simulink model "SimuMCC_LK"  (R2017b)
settings: Solver=VariableStepAuto  StartTime=0.0  StopTime=Tf  MaxStep=1e-4  RelTol=1e-3
values from neighbouring files (symbols this model uses):
  C0 = 0.0    (= 0)    [DataMCCEchant.m]
  Cl = 0    [DataMCCEchant.m]
  F = 0.0001    [DataMCCEchant.m]
  J = 2.20e-4    (= 0.00022)    [DataMCCEchant.m]
  Kelec = -place(Ae,Be,Pole_elec_desiree)    [DataMCCEchant.m]
  Kmeca = place(Am,Bm,Pole_meca_desiree)    [DataMCCEchant.m]
  Kphi = 0.061    [DataMCCEchant.m]
  L = 2.7e-3    (= 0.0027)    [DataMCCEchant.m]
  R = 1.22    [DataMCCEchant.m]
  Ts = 1e-4    (= 0.0001)    [DataMCCEchant.m]
undefined symbols (not defined in the file or in its folder): Cg, Commande, Fg, Gg, Ggi, KPi, KPw, TIi, TIw
settings Model: Creator=romaindelpoux  LastModifiedBy=Lubin Kerhuel
settings SolverCC: ZeroCrossControl=DisableAll

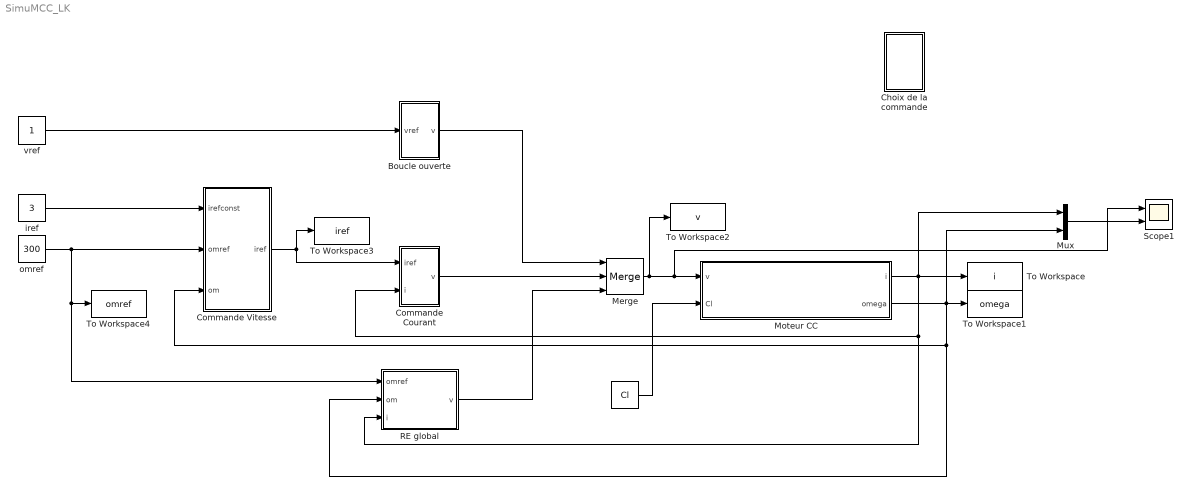
== system SimuMCC_LK ==
  " " : Constant  Value=Cl
  Boucle ouverte : Subsystem
  Choix de la commande : Subsystem
  Commande Courant : Subsystem
  Commande Vitesse : Subsystem
  Merge : Merge  Inputs=3
  Moteur CC : Subsystem
  Mux : Mux  Inputs=2
  RE global : Subsystem
  Scope1 : Scope  NumInputPorts=2
  To Workspace : ToWorkspace  VariableName=i  SaveFormat=Timeseries  SampleTime=-1
  To Workspace1 : ToWorkspace  VariableName=omega  SaveFormat=Timeseries  SampleTime=-1
  To Workspace2 : ToWorkspace  VariableName=v  SaveFormat=Timeseries  SampleTime=-1
  To Workspace3 : ToWorkspace  VariableName=iref  SaveFormat=Timeseries  SampleTime=-1
  To Workspace4 : ToWorkspace  VariableName=omref  SaveFormat=Timeseries  SampleTime=-1
  iref : Constant  Value=3
  omref : Constant  Value=300
  vref : Constant
  wires:
  Merge/1 -> To Workspace2/1, Scope1/1, Moteur CC/1(v)
  Moteur CC/2(omega) -> Mux/2, To Workspace1/1, RE global/2(om), Commande Vitesse/3(om)
  Moteur CC/1(i) -> Mux/1, RE global/3(i), Commande Courant/2(i), To Workspace/1
  omref/1 -> RE global/1(omref), To Workspace4/1, Commande Vitesse/2(omref)
  Commande Courant/1(v) -> Merge/2
  Commande Vitesse/1(iref) -> Commande Courant/1(iref), To Workspace3/1
  " "/1 -> Moteur CC/2(Cl)
  iref/1 -> Commande Vitesse/1(irefconst)
  vref/1 -> Boucle ouverte/1(vref)
  Boucle ouverte/1(v) -> Merge/1
  RE global/1(v) -> Merge/3
  Mux/1 -> Scope1/2

== system SimuMCC_LK/Boucle ouverte ==
  vref : Inport
  BO : Subsystem  TreatAsAtomicUnit=on
  v : Outport
  wires:
  BO/1(v) -> v/1
  vref/1 -> BO/1(vref)
  [BO] -> BO/Action

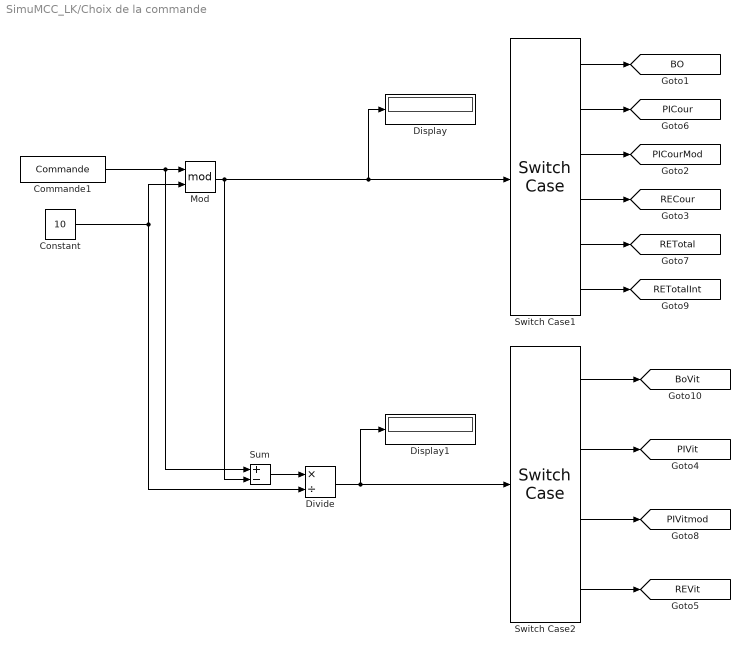
== system SimuMCC_LK/Choix de la commande ==
  Commande1 : Constant  Value=Commande
  Constant : Constant  Value=10
  Display : Display
  Display1 : Display
  Divide : Product  Inputs=*/
  Mod : Math  Operator=mod  SaturateOnIntegerOverflow=on
  Sum : Sum  Inputs=+-
  Switch Case1 : SwitchCase  CaseConditions={0, 1,2,3,4,5}  ShowDefaultCase=off
  Switch Case2 : SwitchCase  CaseConditions={0,1,2,3}  ShowDefaultCase=off
  tag scope: BO=global, BoVit=global, PICour=global, PICourMod=global, PIVit=global, PIVitmod=global, RECour=global, RETotal=global, RETotalInt=global, REVit=global
  wires:
  Switch Case1/1 -> [BO]
  Switch Case1/2 -> [PICour]
  Commande1/1 -> Sum/1, Mod/1
  Switch Case1/3 -> [PICourMod]
  Switch Case1/4 -> [RECour]
  Switch Case2/3 -> [PIVitmod]
  Switch Case2/2 -> [PIVit]
  Switch Case2/1 -> [BoVit]
  Switch Case1/5 -> [RETotal]
  Divide/1 -> Display1/1, Switch Case2/1
  Constant/1 -> Divide/2, Mod/2
  Sum/1 -> Divide/1
  Mod/1 -> Sum/2, Display/1, Switch Case1/1
  Switch Case1/6 -> [RETotalInt]
  Switch Case2/4 -> [REVit]

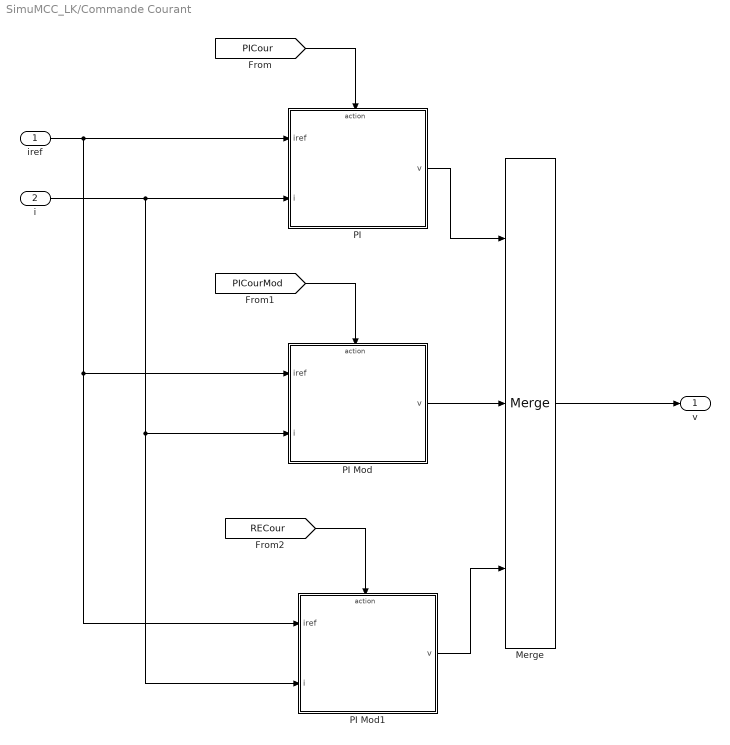
== system SimuMCC_LK/Commande Courant ==
  iref : Inport
  i : Inport  Port=2
  Merge : Merge  Inputs=3
  PI : Subsystem  TreatAsAtomicUnit=on
  PI Mod : Subsystem  TreatAsAtomicUnit=on
  PI Mod1 : Subsystem  TreatAsAtomicUnit=on
  v : Outport
  wires:
  [PICour] -> PI/Action
  iref/1 -> PI Mod/1(iref), PI Mod1/1(iref), PI/1(iref)
  PI/1(v) -> Merge/1
  i/1 -> PI Mod1/2(i), PI Mod/2(i), PI/2(i)
  Merge/1 -> v/1
  PI Mod/1(v) -> Merge/2
  [PICourMod] -> PI Mod/Action
  [RECour] -> PI Mod1/Action
  PI Mod1/1(v) -> Merge/3

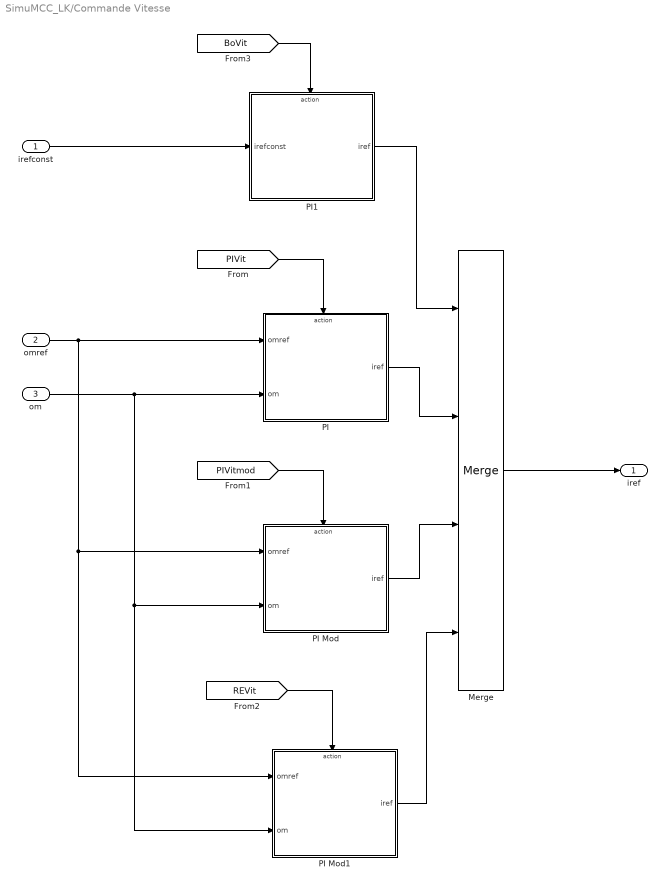
== system SimuMCC_LK/Commande Vitesse ==
  irefconst : Inport
  omref : Inport  Port=2
  om : Inport  Port=3
  Merge : Merge  Inputs=4
  PI : Subsystem  TreatAsAtomicUnit=on
  PI Mod : Subsystem  TreatAsAtomicUnit=on
  PI Mod1 : Subsystem  TreatAsAtomicUnit=on
  PI1 : Subsystem  TreatAsAtomicUnit=on
  iref : Outport
  wires:
  [PIVit] -> PI/Action
  omref/1 -> PI Mod/1(omref), PI Mod1/1(omref), PI/1(omref)
  PI/1(iref) -> Merge/2
  om/1 -> PI Mod/2(om), PI Mod1/2(om), PI/2(om)
  Merge/1 -> iref/1
  PI Mod/1(iref) -> Merge/3
  [PIVitmod] -> PI Mod/Action
  [REVit] -> PI Mod1/Action
  PI Mod1/1(iref) -> Merge/4
  PI1/1(iref) -> Merge/1
  irefconst/1 -> PI1/1(irefconst)
  [BoVit] -> PI1/Action

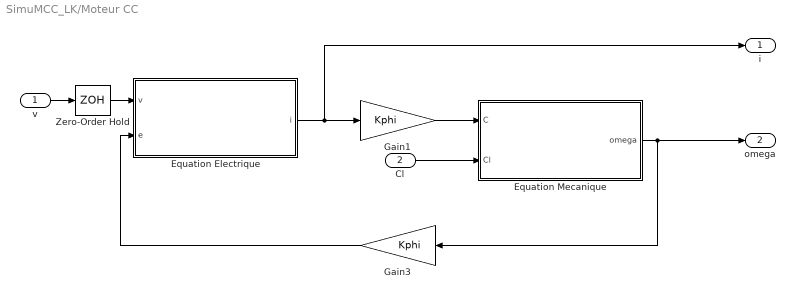
== system SimuMCC_LK/Moteur CC ==
  v : Inport
  Cl : Inport  Port=2
  Equation Electrique : Subsystem
  Equation Mecanique : Subsystem
  Gain1 : Gain  Gain=Kphi
  "Gain3  " : Gain  Gain=Kphi
  Zero-Order Hold : ZeroOrderHold  SampleTime=Ts
  i : Outport
  omega : Outport  Port=2
  wires:
  v/1 -> Zero-Order Hold/1
  "Gain3  "/1 -> Equation Electrique/2(e)
  Gain1/1 -> Equation Mecanique/1(C)
  Cl/1 -> Equation Mecanique/2(Cl)
  Zero-Order Hold/1 -> Equation Electrique/1(v)
  Equation Electrique/1(i) -> i/1, Gain1/1
  Equation Mecanique/1(omega) -> omega/1, "Gain3  "/1

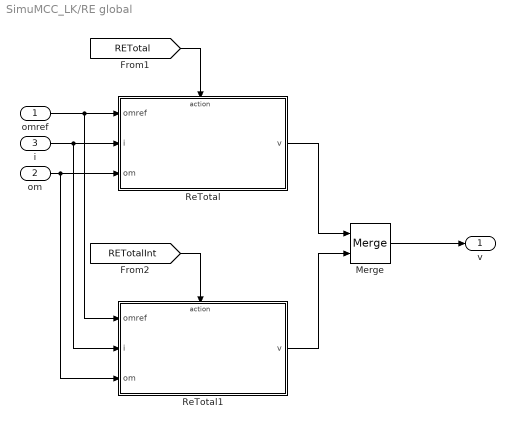
== system SimuMCC_LK/RE global ==
  omref : Inport
  om : Inport  Port=2
  i : Inport  Port=3
  Merge : Merge
  ReTotal : Subsystem  TreatAsAtomicUnit=on
  ReTotal1 : Subsystem  TreatAsAtomicUnit=on
  v : Outport
  wires:
  [RETotal] -> ReTotal/Action
  ReTotal/1(v) -> Merge/1
  om/1 -> ReTotal1/3(" om"), ReTotal/3(" om")
  omref/1 -> ReTotal1/1("omref "), ReTotal/1("omref ")
  [RETotalInt] -> ReTotal1/Action
  i/1 -> ReTotal1/2(" i"), ReTotal/2(" i")
  ReTotal1/1(v) -> Merge/2
  Merge/1 -> v/1

== system SimuMCC_LK/Boucle ouverte/BO ==
  vref : Inport
  Action Port : ActionPort  ActionType=case
  v : Outport
  wires:
  vref/1 -> v/1

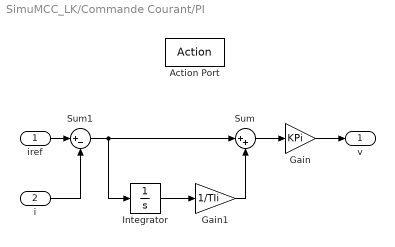
== system SimuMCC_LK/Commande Courant/PI ==
  iref : Inport
  i : Inport  Port=2
  Action Port : ActionPort  ActionType=case
  Gain : Gain  Gain=KPi
  Gain1 : Gain  Gain=1/TIi
  Integrator : Integrator
  Sum : Sum  Inputs=|++
  Sum1 : Sum  Inputs=|+-
  v : Outport
  wires:
  iref/1 -> Sum1/1
  Sum/1 -> Gain/1
  i/1 -> Sum1/2
  Sum1/1 -> Sum/1, Integrator/1
  Gain1/1 -> Sum/2
  Integrator/1 -> Gain1/1
  Gain/1 -> v/1

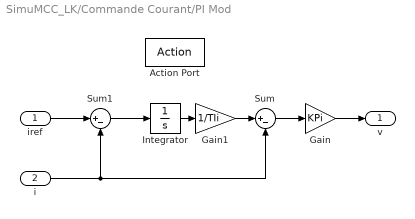
== system SimuMCC_LK/Commande Courant/PI Mod ==
  iref : Inport
  i : Inport  Port=2
  Action Port : ActionPort  ActionType=case
  Gain : Gain  Gain=KPi
  Gain1 : Gain  Gain=1/TIi
  Integrator : Integrator
  Sum : Sum  Inputs=|+-
  Sum1 : Sum  Inputs=|+-
  v : Outport
  wires:
  iref/1 -> Sum1/1
  Sum/1 -> Gain/1
  i/1 -> Sum/2, Sum1/2
  Sum1/1 -> Integrator/1
  Integrator/1 -> Gain1/1
  Gain/1 -> v/1
  Gain1/1 -> Sum/1

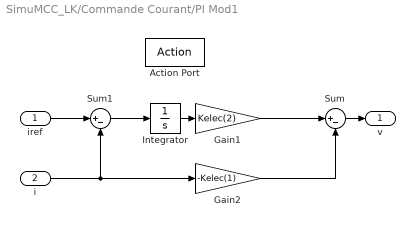
== system SimuMCC_LK/Commande Courant/PI Mod1 ==
  iref : Inport
  i : Inport  Port=2
  Action Port : ActionPort  ActionType=case
  Gain1 : Gain  Gain=Kelec(2)
  Gain2 : Gain  Gain=-Kelec(1)
  Integrator : Integrator
  Sum : Sum  Inputs=|+-
  Sum1 : Sum  Inputs=|+-
  v : Outport
  wires:
  iref/1 -> Sum1/1
  i/1 -> Gain2/1, Sum1/2
  Sum1/1 -> Integrator/1
  Integrator/1 -> Gain1/1
  Sum/1 -> v/1
  Gain1/1 -> Sum/1
  Gain2/1 -> Sum/2

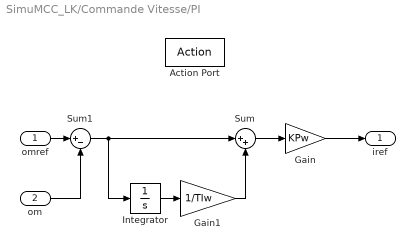
== system SimuMCC_LK/Commande Vitesse/PI ==
  omref : Inport
  om : Inport  Port=2
  Action Port : ActionPort  ActionType=case
  Gain : Gain  Gain=KPw
  Gain1 : Gain  Gain=1/TIw
  Integrator : Integrator
  Sum : Sum  Inputs=|++
  Sum1 : Sum  Inputs=|+-
  iref : Outport
  wires:
  omref/1 -> Sum1/1
  Sum/1 -> Gain/1
  om/1 -> Sum1/2
  Sum1/1 -> Sum/1, Integrator/1
  Gain1/1 -> Sum/2
  Integrator/1 -> Gain1/1
  Gain/1 -> iref/1

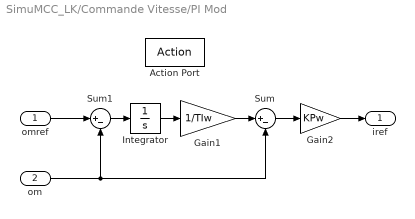
== system SimuMCC_LK/Commande Vitesse/PI Mod ==
  omref : Inport
  om : Inport  Port=2
  Action Port : ActionPort  ActionType=case
  Gain1 : Gain  Gain=1/TIw
  Gain2 : Gain  Gain=KPw
  Integrator : Integrator
  Sum : Sum  Inputs=|+-
  Sum1 : Sum  Inputs=|+-
  iref : Outport
  wires:
  omref/1 -> Sum1/1
  Sum/1 -> Gain2/1
  om/1 -> Sum/2, Sum1/2
  Sum1/1 -> Integrator/1
  Gain2/1 -> iref/1
  Gain1/1 -> Sum/1
  Integrator/1 -> Gain1/1

== system SimuMCC_LK/Commande Vitesse/PI Mod1 ==
  omref : Inport
  om : Inport  Port=2
  Action Port : ActionPort  ActionType=case
  Gain1 : Gain  Gain=Kmeca(2)
  Gain2 : Gain  Gain=Kmeca(1)
  Integrator : Integrator
  Sum : Sum  Inputs=|--
  Sum1 : Sum  Inputs=|+-
  iref : Outport
  wires:
  omref/1 -> Sum1/1
  om/1 -> Gain2/1, Sum1/2
  Sum1/1 -> Integrator/1
  Integrator/1 -> Gain1/1
  Sum/1 -> iref/1
  Gain1/1 -> Sum/1
  Gain2/1 -> Sum/2

== system SimuMCC_LK/Commande Vitesse/PI1 ==
  irefconst : Inport
  Action Port : ActionPort  ActionType=case
  iref : Outport
  wires:
  irefconst/1 -> iref/1

== system SimuMCC_LK/Moteur CC/Equation Electrique ==
  v : Inport
  e : Inport  Port=2
  Gain : Gain  Gain=1/L
  Gain1 : Gain  Gain=R
  Integrator : Integrator
  Sum : Sum  Inputs=+--
  i : Outport
  wires:
  Gain1/1 -> Sum/2
  Sum/1 -> Gain/1
  Integrator/1 -> i/1, Gain1/1  "i"
  Gain/1 -> Integrator/1  "di"
  v/1 -> Sum/1
  e/1 -> Sum/3

== system SimuMCC_LK/Moteur CC/Equation Mecanique ==
  C : Inport
  Cl : Inport  Port=2
  Gain : Gain  Gain=1/J
  Gain1 : Gain  Gain=F
  Gain2 : Gain  Gain=C0
  Integrator : Integrator
  Sign : Signum
  Sum : Sum  Inputs=+-+-
  omega : Outport
  wires:
  Gain/1 -> Integrator/1  "domega"
  Integrator/1 -> Sign/1, Gain1/1, omega/1  "omega"
  Sum/1 -> Gain/1
  Gain1/1 -> Sum/2
  Sign/1 -> Gain2/1
  Gain2/1 -> Sum/3
  C/1 -> Sum/1
  Cl/1 -> Sum/4

== system SimuMCC_LK/RE global/ReTotal ==
  "omref " : Inport
  " i" : Inport  Port=2
  " om" : Inport  Port=3
  Action Port : ActionPort  ActionType=case
  Gain : Gain  Gain=Gg  Multiplication=Matrix(K*u)
  Gain1 : Gain  Gain=Fg  Multiplication=Matrix(K*u)
  Mux : Mux  Inputs=2
  Sum : Sum  Inputs=|-+
  v : Outport
  wires:
  " om"/1 -> Mux/2
  " i"/1 -> Mux/1
  Mux/1 -> Gain/1
  Gain/1 -> Sum/1
  Sum/1 -> v/1
  "omref "/1 -> Gain1/1
  Gain1/1 -> Sum/2

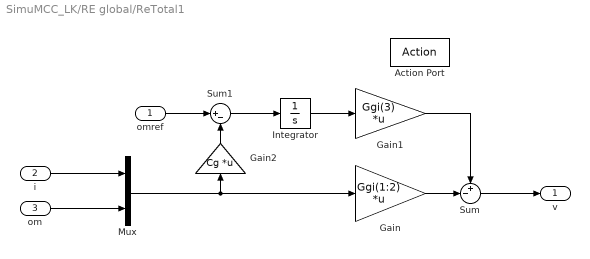
== system SimuMCC_LK/RE global/ReTotal1 ==
  "omref " : Inport
  " i" : Inport  Port=2
  " om" : Inport  Port=3
  Action Port : ActionPort  ActionType=case
  Gain : Gain  Gain=Ggi(1:2)  Multiplication=Matrix(K*u)
  Gain1 : Gain  Gain=Ggi(3)  Multiplication=Matrix(K*u)
  Gain2 : Gain  Gain=Cg  Multiplication=Matrix(K*u)
  Integrator : Integrator
  Mux : Mux  Inputs=2
  Sum : Sum  Inputs=+-|
  Sum1 : Sum  Inputs=|+-
  v : Outport
  wires:
  Gain1/1 -> Sum/1
  "omref "/1 -> Sum1/1
  Sum/1 -> v/1
  Gain/1 -> Sum/2
  Mux/1 -> Gain/1, Gain2/1
  " i"/1 -> Mux/1
  " om"/1 -> Mux/2
  Sum1/1 -> Integrator/1
  Gain2/1 -> Sum1/2
  Integrator/1 -> Gain1/1
